simulink model "tf_model"  (R2021b)
settings: Solver=ode4  StartTime=0.0  StopTime=0.001  FixedStep=0.001  RelTol=1e-3
settings Model: Creator=valeriytashchilin  LastModifiedBy=valeriytashchilin
settings DataIOCC: LoadInitialState=on  SaveFinalState=on  SaveFormat=StructureWithTime  SignalLogging=off  DSMLogging=off  SaveTime=off  ReturnWorkspaceOutputs=off

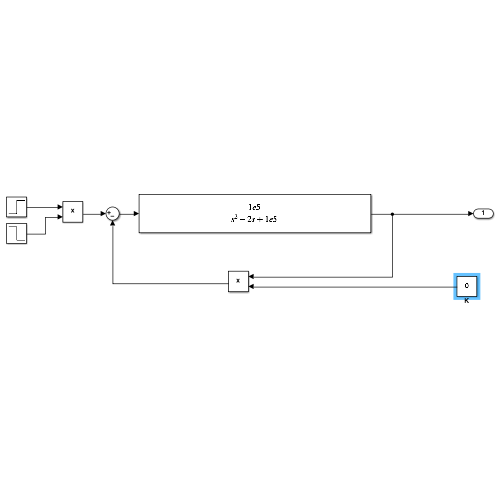
[thumbnail: Simulink's stored preview of the top-level diagram]
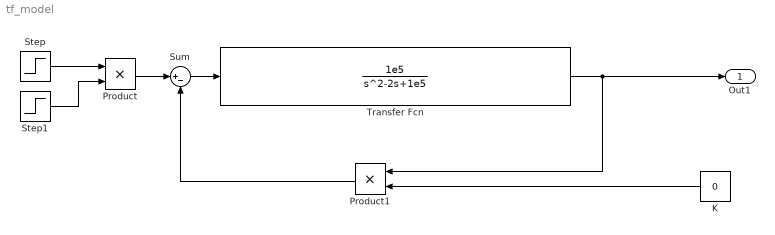
== system tf_model ==
  K : Constant  Value=0
  Product : Product
  Product1 : Product
  Step : Step  Time=0.1  SampleTime=0
  Step1 : Step  Time=0.11  Before=1  After=0  SampleTime=0
  Sum : Sum  Inputs=|+-
  Transfer Fcn : TransferFcn  Numerator=[1e5]  Denominator=[1, -2, 1e5]
  Out1 : Outport
  wires:
  Step/1 -> Product/1
  Step1/1 -> Product/2
  Transfer Fcn/1 -> Out1/1, Product1/1
  Product/1 -> Sum/1
  Sum/1 -> Transfer Fcn/1
  Product1/1 -> Sum/2
  K/1 -> Product1/2
